simulink model "problem2"  (R2020a)
settings: Solver=VariableStepAuto  StartTime=0.0  StopTime=100  RelTol=1e-3
model workspace (MAT data in the model file):
  K1 = 50
  K2 = 30
  M1 = 100
  M2 = 120
  b = 50
settings Model: Creator=kasutav  LastModifiedBy=kasutav
settings DataIOCC: ExternalInput=[th, br]

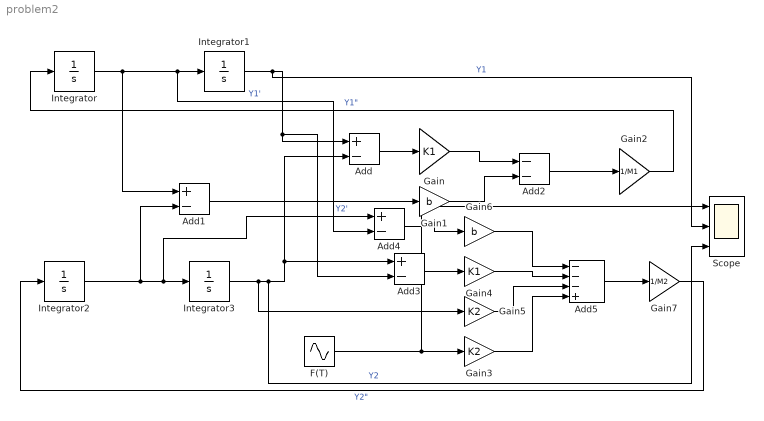
== system problem2 ==
  Add{,1,3..4} (4 alike) : Sum  Inputs=+-
  Add2 : Sum  Inputs=--
  Add5 : Sum  Inputs=---+
  F(T) : Sin  SampleTime=0
  Gain : Gain  Gain=K1
  Gain1 : Gain  Gain=b
  Gain2 : Gain  Gain=1/M1
  Gain3 : Gain  Gain=K2
  Gain4 : Gain  Gain=K1
  Gain5 : Gain  Gain=K2
  Gain6 : Gain  Gain=b
  Gain7 : Gain  Gain=1/M2
  Integrator{,1..3} (4 alike) : Integrator
  Scope : Scope  NumInputPorts=3
  wires:
  Gain2/1 -> Integrator/1  "Y1\""
  Integrator/1 -> Add1/1, Add4/2, Integrator1/1  "Y1'"
  Integrator1/1 -> Scope/2, Add3/2, Add/1  "Y1"
  Integrator2/1 -> Add1/2, Add4/1, Integrator3/1  "Y2'"
  Gain7/1 -> Integrator2/1  "Y2\""
  Integrator3/1 -> Gain5/1, Scope/3, Add3/1, Add/2  "Y2"
  Add/1 -> Gain/1
  Add1/1 -> Gain1/1
  Gain/1 -> Add2/1
  Gain1/1 -> Add2/2
  Add2/1 -> Gain2/1
  F(T)/1 -> Gain3/1, Scope/1
  Add3/1 -> Gain4/1
  Add4/1 -> Gain6/1
  Gain3/1 -> Add5/4
  Gain5/1 -> Add5/3
  Gain4/1 -> Add5/2
  Gain6/1 -> Add5/1
  Add5/1 -> Gain7/1
